simulink model "gm_inc_enc_v26_vnl"  (R2022b)
settings: Solver=FixedStepDiscrete  StartTime=0.0  StopTime=SimulationsDauer  RelTol=1e-3
undefined symbols (not defined in the file or in its folder): CW_CCW_Switch, d_axis_hit_CompareValue, DiscIntNeverNeededParam, f_ISR, IncPerTurn, inital_zero_speed_timeout, n_max, Offset_Position_elec, Offset_Position_mech, OmegaPerOverSampl, Periode, Phase_Delay_A, Phase_Delay_B, PolePair, QuadratureFactor, reciprocal_iterations, T_fpga, T_mech
libraries: simulink x25, hdlsllib x11, hdlmdlgenlib x4, dspsrcs4 x3, dspswit3 x2, spsEdgeDetectorLib x2, simulink_extras x1
(part 4 of 5)

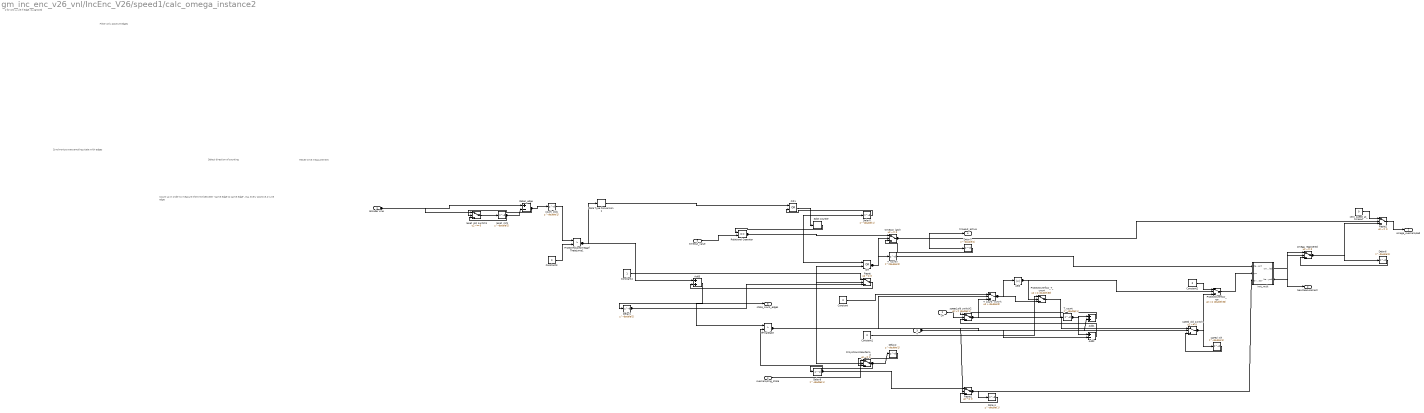
== system gm_inc_enc_v26_vnl/IncEnc_V26/speed1/calc_omega_instance2 ==
  note: Synchronize oversampling state with edges
  note: Filter only positive edges
  note: Select direction of counting
  note: 1 for one cycle if edge recognized
  note: Reset time measurement
  note: Count up in order to measure the time between "same edge to same edge", e.g. every positive A-Line edge
  Encoder Line : Inport  OutDataTypeStr=boolean  PortDimensions=1  SampleTime=1e-08
  Dir : Inport  Port=2  OutDataTypeStr=fixdt(1, 4, 0)  PortDimensions=1  SampleTime=1e-08
  T : Inport  Port=3  OutDataTypeStr=fixdt(1, 38, 32)  PortDimensions=1  SampleTime=1e-08
  oversampling_state : Inport  Port=4  OutDataTypeStr=uint16  PortDimensions=1  SampleTime=1e-08
  timeout_value : Inport  Port=5  OutDataTypeStr=uint32  PortDimensions=1  SampleTime=1e-08
  32bit counter : hdlsllib/Sources/HDL Counter  CountType=Free running  CountInit=0  CountStep=1  CountMax=inital_zero_speed_timeout  CountFromType=Initial value  CountFrom=0  CountResetPort=on  CountLoadPort=off  CountEnbPort=off  CountDirPort=off  CountHitOutputPort=off  CountDataType=Unsigned  CountWordLen=32  CountFracLen=0  CountSampTime=1
  ABS : Abs  SampleTime=1e-08  OutDataTypeStr=fixdt(1, 38, 32)  SaturateOnIntegerOverflow=off
  Add1 : Sum  AccumDataTypeStr=fixdt(1, 38, 32)  OutDataTypeStr=fixdt(1, 38, 32)  SampleTime=1e-08
  Add2 : Sum  Inputs=+-  AccumDataTypeStr=fixdt(1, 38, 32)  OutDataTypeStr=fixdt(1, 38, 32)  SampleTime=1e-08
  Add3 : Sum  AccumDataTypeStr=int16  OutDataTypeStr=int16  SampleTime=1e-08
  Constant : Constant  Value=0  OutDataTypeStr=fixdt(1, 38, 32)  SampleTime=1e-08
  Constant1 : Constant  Value=0  OutDataTypeStr=fixdt(1, 38, 32)  SampleTime=1e-08
  Constant2 : Constant  Value=0  OutDataTypeStr=fixdt(1, 38, 32)  SampleTime=1e-08
  Constant3 : Constant  Value=0  OutDataTypeStr=int8  SampleTime=1e-08
  Constant4 : Constant  OutDataTypeStr=int8  SampleTime=1e-08
  Data Type Conversion1 : DataTypeConversion  OutDataTypeStr=boolean  SampleTime=1e-08  SaturateOnIntegerOverflow=off  RndMeth=Floor
  Delay{1..6,8} (7 alike) : Delay  DelayLength=double(1)  InitialCondition=0  SampleTime=1e-08
  Detec_edge : Sum  Inputs=+-  AccumDataTypeStr=int8  OutDataTypeStr=int8  SampleTime=1e-08
  IfFinalState : RelationalOperator  Operator=>  OutDataTypeStr=boolean  SampleTime=1e-08  InputSameDT=off
  OR : Logic  Operator=OR  AllPortsSameDT=off  OutDataTypeStr=boolean  SampleTime=1e-08
  OR1 : Logic  Operator=OR  AllPortsSameDT=off  OutDataTypeStr=boolean  SampleTime=1e-08
  OnlyAllowInNewPeriod : Switch  Criteria=u2 ~= 0  Threshold=double(0)  OutDataTypeStr=uint16  SampleTime=1e-08  SaturateOnIntegerOverflow=off  InputSameDT=off
  ProtectOverflow_T_count : Switch  Threshold=double(30)  OutDataTypeStr=fixdt(1, 38, 32)  SampleTime=1e-08  SaturateOnIntegerOverflow=off  InputSameDT=off
  ProtectOverflow_rps : Switch  Threshold=double(30)  OutDataTypeStr=fixdt(1, 38, 32)  SampleTime=1e-08  SaturateOnIntegerOverflow=off  InputSameDT=off
  ProtectToUseOmegaIfThetaJump1 : RelationalOperator  Operator=>  OutDataTypeStr=fixdt(1,16,0)  SampleTime=1e-08  InputSameDT=off
  Relational Operator : RelationalOperator  Operator===  OutDataTypeStr=boolean  SampleTime=1e-08  InputSameDT=off
  Reset : Switch  Criteria=u2 ~= 0  Threshold=double(0)  OutDataTypeStr=fixdt(1, 24, 11)  SampleTime=1e-08  SaturateOnIntegerOverflow=off  InputSameDT=off
  Reset1 : Switch  Criteria=u2 ~= 0  Threshold=double(0)  OutDataTypeStr=uint16  SampleTime=1e-08  SaturateOnIntegerOverflow=off  InputSameDT=off
  Reset2 : Switch  Criteria=u2 ~= 0  Threshold=double(0)  OutDataTypeStr=fixdt(1, 24, 11)  SampleTime=1e-08  SaturateOnIntegerOverflow=off  InputSameDT=off
  T_count : Delay  DelayLength=double(1)  InitialCondition=0  SampleTime=1e-08
  T_count1 : Delay  DelayLength=double(2)  InitialCondition=0  SampleTime=1e-08
  T_count_switch : Switch  Criteria=u2 > Threshold  Threshold=double(0)  OutDataTypeStr=fixdt(1, 38, 32)  SampleTime=1e-08  SaturateOnIntegerOverflow=off  InputSameDT=off
  count_old1 : Delay  DelayLength=double(1)  InitialCondition=0  SampleTime=1e-08
  invt_mult : Subsystem
  omega_registered : Switch  Criteria=u2 ~= 0  Threshold=double(0)  OutDataTypeStr=fixdt(1, 24, 11)  SampleTime=1e-08  SaturateOnIntegerOverflow=off  InputSameDT=off
  reset_old1 : Delay  DelayLength=double(1)  InitialCondition=0  SampleTime=1e-08
  reset_old_switch1 : Switch  Criteria=u2 ~= 0  Threshold=double(0)  OutDataTypeStr=boolean  SampleTime=1e-08  SaturateOnIntegerOverflow=off  InputSameDT=off
  speed_old : Delay  DelayLength=double(1)  InitialCondition=0  SampleTime=1e-08
  speed_old_switch : Switch  Criteria=u2 ~= 0  Threshold=double(0)  OutDataTypeStr=fixdt(1, 38, 32)  SampleTime=1e-08  SaturateOnIntegerOverflow=off  InputSameDT=off
  speed_old_switch2 : Switch  Threshold=double(1)  OutDataTypeStr=fixdt(1, 38, 32)  SampleTime=1e-08  SaturateOnIntegerOverflow=off  InputSameDT=off
  timeout_latch : Switch  Criteria=u2 ~= 0  Threshold=double(0)  OutDataTypeStr=boolean  SampleTime=1e-08  SaturateOnIntegerOverflow=off  InputSameDT=off
  zero_speed_at_timeout : Constant  Value=0  OutDataTypeStr=fixdt(1, 24, 11)  SampleTime=1e-08
  omega_oversampled : Outport  SampleTime=1e-08  VectorParamsAs1DForOutWhenUnconnected=off
  NewMeasurement : Outport  Port=2  SampleTime=1e-08  VectorParamsAs1DForOutWhenUnconnected=off
  state_count_edges : Outport  Port=3  SampleTime=1e-08  VectorParamsAs1DForOutWhenUnconnected=off
  timeout_active : Outport  Port=4  OutDataTypeStr=boolean  SampleTime=1e-08  VectorParamsAs1DForOutWhenUnconnected=off
  wires:
  Encoder Line/1 -> Detec_edge/1, reset_old_switch1/1
  Dir/1 -> speed_old_switch2/2
  T/1 -> Add1/2, Add2/2
  oversampling_state/1 -> OnlyAllowInNewPeriod/1
  timeout_value/1 -> Relational Operator/2
  zero_speed_at_timeout/1 -> Reset2/1
  timeout_latch/1 -> Reset2/2, timeout_active/1, Delay3/1
  speed_old_switch2/1 -> T_count_switch/3, speed_old_switch/1
  speed_old_switch/1 -> ProtectOverflow_rps/3, speed_old/1
  omega_registered/1 -> Reset2/3, Delay6/1
  invt_mult/1(omega_oversampled) -> omega_registered/1
  invt_mult/2(New_Measurement_delayed) -> NewMeasurement/1, omega_registered/2
  count_old1/1 -> ProtectToUseOmegaIfThetaJump1/1
  T_count1/1 -> invt_mult/1(New_Measurement)
  Reset2/1 -> omega_oversampled/1
  Reset1/1 -> invt_mult/3(Oversampling Factor), Delay4/1
  Relational Operator/1 -> OR/1, Delay5/1, timeout_latch/1
  ProtectToUseOmegaIfThetaJump1/1 -> Data Type Conversion1/1, Add3/1
  ProtectOverflow_rps/1 -> invt_mult/2(rps)
  OR/1 -> T_count1/1, timeout_latch/2
  IfFinalState/1 -> OR/2, OnlyAllowInNewPeriod/2, Reset/2, T_count_switch/2, speed_old_switch/2, Reset1/2
  Detec_edge/1 -> count_old1/1, reset_old_switch1/2
  Delay8/1 -> IfFinalState/2, Reset1/1
  Delay1/1 -> state_count_edges/1, IfFinalState/1, Reset/3
  Data Type Conversion1/1 -> OR1/1
  Constant4/1 -> Reset/1
  Constant3/1 -> ProtectToUseOmegaIfThetaJump1/2
  Constant2/1 -> ProtectOverflow_rps/1
  Constant1/1 -> ProtectOverflow_T_count/1
  Constant/1 -> T_count_switch/1
  ABS/1 -> ProtectOverflow_rps/2, ProtectOverflow_T_count/2
  Delay6/1 -> omega_registered/3
  reset_old_switch1/1 -> reset_old1/1
  reset_old1/1 -> Detec_edge/2, reset_old_switch1/3
  OR1/1 -> 32bit counter/1
  Delay5/1 -> OR1/2
  32bit counter/1 -> Relational Operator/1
  Delay2/1 -> OnlyAllowInNewPeriod/3
  OnlyAllowInNewPeriod/1 -> Delay2/1, Delay8/1
  Reset/1 -> Add3/2
  Add3/1 -> Delay1/1
  Delay3/1 -> timeout_latch/3
  Add2/1 -> speed_old_switch2/3
  ProtectOverflow_T_count/1 -> T_count/1
  T_count/1 -> Add1/1, Add2/1
  Add1/1 -> speed_old_switch2/1
  T_count_switch/1 -> ABS/1, ProtectOverflow_T_count/3
  speed_old/1 -> speed_old_switch/3
  Delay4/1 -> Reset1/3

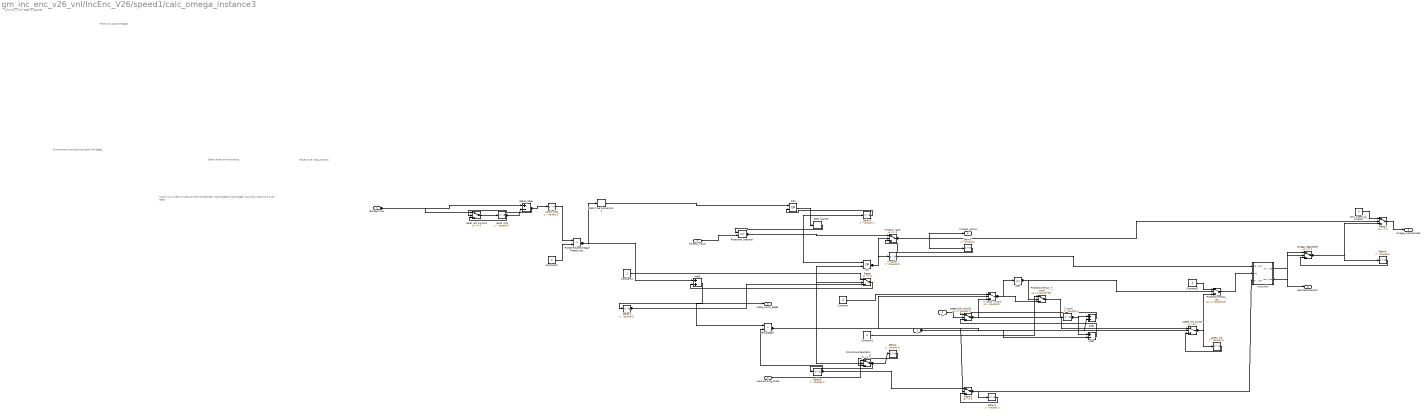
== system gm_inc_enc_v26_vnl/IncEnc_V26/speed1/calc_omega_instance3 ==
  note: Synchronize oversampling state with edges
  note: Filter only positive edges
  note: Select direction of counting
  note: 1 for one cycle if edge recognized
  note: Reset time measurement
  note: Count up in order to measure the time between "same edge to same edge", e.g. every positive A-Line edge
  Encoder Line : Inport  OutDataTypeStr=boolean  PortDimensions=1  SampleTime=1e-08
  Dir : Inport  Port=2  OutDataTypeStr=fixdt(1, 4, 0)  PortDimensions=1  SampleTime=1e-08
  T : Inport  Port=3  OutDataTypeStr=fixdt(1, 38, 32)  PortDimensions=1  SampleTime=1e-08
  oversampling_state : Inport  Port=4  OutDataTypeStr=uint16  PortDimensions=1  SampleTime=1e-08
  timeout_value : Inport  Port=5  OutDataTypeStr=uint32  PortDimensions=1  SampleTime=1e-08
  32bit counter : hdlsllib/Sources/HDL Counter  CountType=Free running  CountInit=0  CountStep=1  CountMax=inital_zero_speed_timeout  CountFromType=Initial value  CountFrom=0  CountResetPort=on  CountLoadPort=off  CountEnbPort=off  CountDirPort=off  CountHitOutputPort=off  CountDataType=Unsigned  CountWordLen=32  CountFracLen=0  CountSampTime=1
  ABS : Abs  SampleTime=1e-08  OutDataTypeStr=fixdt(1, 38, 32)  SaturateOnIntegerOverflow=off
  Add1 : Sum  AccumDataTypeStr=fixdt(1, 38, 32)  OutDataTypeStr=fixdt(1, 38, 32)  SampleTime=1e-08
  Add2 : Sum  Inputs=+-  AccumDataTypeStr=fixdt(1, 38, 32)  OutDataTypeStr=fixdt(1, 38, 32)  SampleTime=1e-08
  Add3 : Sum  AccumDataTypeStr=int16  OutDataTypeStr=int16  SampleTime=1e-08
  Constant : Constant  Value=0  OutDataTypeStr=fixdt(1, 38, 32)  SampleTime=1e-08
  Constant1 : Constant  Value=0  OutDataTypeStr=fixdt(1, 38, 32)  SampleTime=1e-08
  Constant2 : Constant  Value=0  OutDataTypeStr=fixdt(1, 38, 32)  SampleTime=1e-08
  Constant3 : Constant  Value=0  OutDataTypeStr=int8  SampleTime=1e-08
  Constant4 : Constant  OutDataTypeStr=int8  SampleTime=1e-08
  Data Type Conversion1 : DataTypeConversion  OutDataTypeStr=boolean  SampleTime=1e-08  SaturateOnIntegerOverflow=off  RndMeth=Floor
  Delay{1..6,8} (7 alike) : Delay  DelayLength=double(1)  InitialCondition=0  SampleTime=1e-08
  Detec_edge : Sum  Inputs=+-  AccumDataTypeStr=int8  OutDataTypeStr=int8  SampleTime=1e-08
  IfFinalState : RelationalOperator  Operator=>  OutDataTypeStr=boolean  SampleTime=1e-08  InputSameDT=off
  OR : Logic  Operator=OR  AllPortsSameDT=off  OutDataTypeStr=boolean  SampleTime=1e-08
  OR1 : Logic  Operator=OR  AllPortsSameDT=off  OutDataTypeStr=boolean  SampleTime=1e-08
  OnlyAllowInNewPeriod : Switch  Criteria=u2 ~= 0  Threshold=double(0)  OutDataTypeStr=uint16  SampleTime=1e-08  SaturateOnIntegerOverflow=off  InputSameDT=off
  ProtectOverflow_T_count : Switch  Threshold=double(30)  OutDataTypeStr=fixdt(1, 38, 32)  SampleTime=1e-08  SaturateOnIntegerOverflow=off  InputSameDT=off
  ProtectOverflow_rps : Switch  Threshold=double(30)  OutDataTypeStr=fixdt(1, 38, 32)  SampleTime=1e-08  SaturateOnIntegerOverflow=off  InputSameDT=off
  ProtectToUseOmegaIfThetaJump1 : RelationalOperator  Operator=>  OutDataTypeStr=fixdt(1,16,0)  SampleTime=1e-08  InputSameDT=off
  Relational Operator : RelationalOperator  Operator===  OutDataTypeStr=boolean  SampleTime=1e-08  InputSameDT=off
  Reset : Switch  Criteria=u2 ~= 0  Threshold=double(0)  OutDataTypeStr=fixdt(1, 24, 11)  SampleTime=1e-08  SaturateOnIntegerOverflow=off  InputSameDT=off
  Reset1 : Switch  Criteria=u2 ~= 0  Threshold=double(0)  OutDataTypeStr=uint16  SampleTime=1e-08  SaturateOnIntegerOverflow=off  InputSameDT=off
  Reset2 : Switch  Criteria=u2 ~= 0  Threshold=double(0)  OutDataTypeStr=fixdt(1, 24, 11)  SampleTime=1e-08  SaturateOnIntegerOverflow=off  InputSameDT=off
  T_count : Delay  DelayLength=double(1)  InitialCondition=0  SampleTime=1e-08
  T_count1 : Delay  DelayLength=double(2)  InitialCondition=0  SampleTime=1e-08
  T_count_switch : Switch  Criteria=u2 > Threshold  Threshold=double(0)  OutDataTypeStr=fixdt(1, 38, 32)  SampleTime=1e-08  SaturateOnIntegerOverflow=off  InputSameDT=off
  count_old1 : Delay  DelayLength=double(1)  InitialCondition=0  SampleTime=1e-08
  invt_mult : Subsystem
  omega_registered : Switch  Criteria=u2 ~= 0  Threshold=double(0)  OutDataTypeStr=fixdt(1, 24, 11)  SampleTime=1e-08  SaturateOnIntegerOverflow=off  InputSameDT=off
  reset_old1 : Delay  DelayLength=double(1)  InitialCondition=0  SampleTime=1e-08
  reset_old_switch1 : Switch  Criteria=u2 ~= 0  Threshold=double(0)  OutDataTypeStr=boolean  SampleTime=1e-08  SaturateOnIntegerOverflow=off  InputSameDT=off
  speed_old : Delay  DelayLength=double(1)  InitialCondition=0  SampleTime=1e-08
  speed_old_switch : Switch  Criteria=u2 ~= 0  Threshold=double(0)  OutDataTypeStr=fixdt(1, 38, 32)  SampleTime=1e-08  SaturateOnIntegerOverflow=off  InputSameDT=off
  speed_old_switch2 : Switch  Threshold=double(1)  OutDataTypeStr=fixdt(1, 38, 32)  SampleTime=1e-08  SaturateOnIntegerOverflow=off  InputSameDT=off
  timeout_latch : Switch  Criteria=u2 ~= 0  Threshold=double(0)  OutDataTypeStr=boolean  SampleTime=1e-08  SaturateOnIntegerOverflow=off  InputSameDT=off
  zero_speed_at_timeout : Constant  Value=0  OutDataTypeStr=fixdt(1, 24, 11)  SampleTime=1e-08
  omega_oversampled : Outport  SampleTime=1e-08  VectorParamsAs1DForOutWhenUnconnected=off
  NewMeasurement : Outport  Port=2  SampleTime=1e-08  VectorParamsAs1DForOutWhenUnconnected=off
  state_count_edges : Outport  Port=3  SampleTime=1e-08  VectorParamsAs1DForOutWhenUnconnected=off
  timeout_active : Outport  Port=4  OutDataTypeStr=boolean  SampleTime=1e-08  VectorParamsAs1DForOutWhenUnconnected=off
  wires:
  Encoder Line/1 -> Detec_edge/1, reset_old_switch1/1
  Dir/1 -> speed_old_switch2/2
  T/1 -> Add1/2, Add2/2
  oversampling_state/1 -> OnlyAllowInNewPeriod/1
  timeout_value/1 -> Relational Operator/2
  zero_speed_at_timeout/1 -> Reset2/1
  timeout_latch/1 -> Reset2/2, timeout_active/1, Delay3/1
  speed_old_switch2/1 -> T_count_switch/3, speed_old_switch/1
  speed_old_switch/1 -> ProtectOverflow_rps/3, speed_old/1
  omega_registered/1 -> Reset2/3, Delay6/1
  invt_mult/1(omega_oversampled) -> omega_registered/1
  invt_mult/2(New_Measurement_delayed) -> NewMeasurement/1, omega_registered/2
  count_old1/1 -> ProtectToUseOmegaIfThetaJump1/1
  T_count1/1 -> invt_mult/1(New_Measurement)
  Reset2/1 -> omega_oversampled/1
  Reset1/1 -> invt_mult/3(Oversampling Factor), Delay4/1
  Relational Operator/1 -> OR/1, Delay5/1, timeout_latch/1
  ProtectToUseOmegaIfThetaJump1/1 -> Data Type Conversion1/1, Add3/1
  ProtectOverflow_rps/1 -> invt_mult/2(rps)
  OR/1 -> T_count1/1, timeout_latch/2
  IfFinalState/1 -> OR/2, OnlyAllowInNewPeriod/2, Reset/2, T_count_switch/2, speed_old_switch/2, Reset1/2
  Detec_edge/1 -> count_old1/1, reset_old_switch1/2
  Delay8/1 -> IfFinalState/2, Reset1/1
  Delay1/1 -> state_count_edges/1, IfFinalState/1, Reset/3
  Data Type Conversion1/1 -> OR1/1
  Constant4/1 -> Reset/1
  Constant3/1 -> ProtectToUseOmegaIfThetaJump1/2
  Constant2/1 -> ProtectOverflow_rps/1
  Constant1/1 -> ProtectOverflow_T_count/1
  Constant/1 -> T_count_switch/1
  ABS/1 -> ProtectOverflow_rps/2, ProtectOverflow_T_count/2
  Delay6/1 -> omega_registered/3
  reset_old_switch1/1 -> reset_old1/1
  reset_old1/1 -> Detec_edge/2, reset_old_switch1/3
  OR1/1 -> 32bit counter/1
  Delay5/1 -> OR1/2
  32bit counter/1 -> Relational Operator/1
  Delay2/1 -> OnlyAllowInNewPeriod/3
  OnlyAllowInNewPeriod/1 -> Delay2/1, Delay8/1
  Reset/1 -> Add3/2
  Add3/1 -> Delay1/1
  Delay3/1 -> timeout_latch/3
  Add2/1 -> speed_old_switch2/3
  ProtectOverflow_T_count/1 -> T_count/1
  T_count/1 -> Add1/1, Add2/1
  Add1/1 -> speed_old_switch2/1
  T_count_switch/1 -> ABS/1, ProtectOverflow_T_count/3
  speed_old/1 -> speed_old_switch/3
  Delay4/1 -> Reset1/3

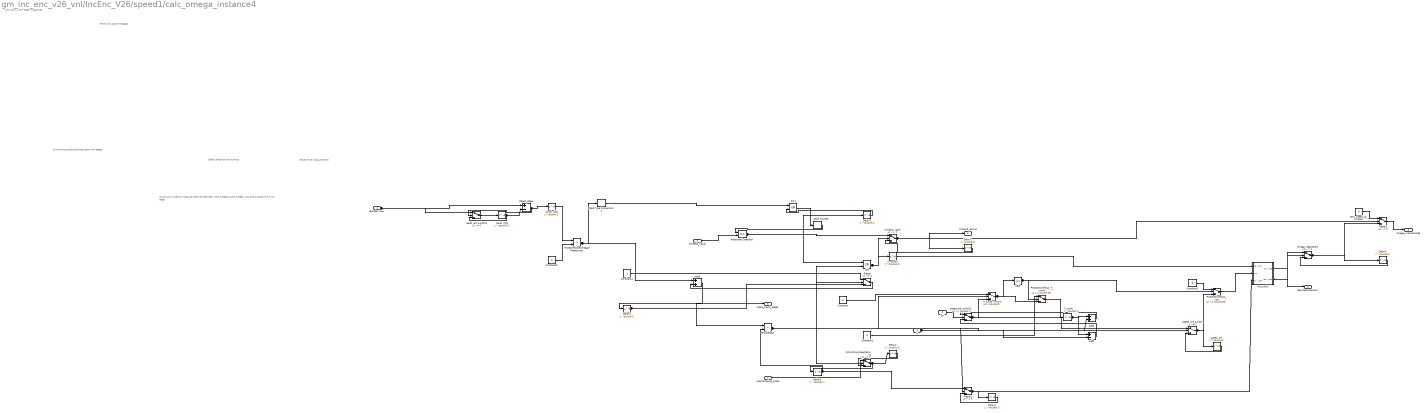
== system gm_inc_enc_v26_vnl/IncEnc_V26/speed1/calc_omega_instance4 ==
  note: Count up in order to measure the time between "same edge to same edge", e.g. every positive A-Line edge
  note: Reset time measurement
  note: 1 for one cycle if edge recognized
  note: Select direction of counting
  note: Filter only positive edges
  note: Synchronize oversampling state with edges
  Encoder Line : Inport  OutDataTypeStr=boolean  PortDimensions=1  SampleTime=1e-08
  Dir : Inport  Port=2  OutDataTypeStr=fixdt(1, 4, 0)  PortDimensions=1  SampleTime=1e-08
  T : Inport  Port=3  OutDataTypeStr=fixdt(1, 38, 32)  PortDimensions=1  SampleTime=1e-08
  oversampling_state : Inport  Port=4  OutDataTypeStr=uint16  PortDimensions=1  SampleTime=1e-08
  timeout_value : Inport  Port=5  OutDataTypeStr=uint32  PortDimensions=1  SampleTime=1e-08
  32bit counter : hdlsllib/Sources/HDL Counter  CountType=Free running  CountInit=0  CountStep=1  CountMax=inital_zero_speed_timeout  CountFromType=Initial value  CountFrom=0  CountResetPort=on  CountLoadPort=off  CountEnbPort=off  CountDirPort=off  CountHitOutputPort=off  CountDataType=Unsigned  CountWordLen=32  CountFracLen=0  CountSampTime=1
  ABS : Abs  SampleTime=1e-08  OutDataTypeStr=fixdt(1, 38, 32)  SaturateOnIntegerOverflow=off
  Add1 : Sum  AccumDataTypeStr=fixdt(1, 38, 32)  OutDataTypeStr=fixdt(1, 38, 32)  SampleTime=1e-08
  Add2 : Sum  Inputs=+-  AccumDataTypeStr=fixdt(1, 38, 32)  OutDataTypeStr=fixdt(1, 38, 32)  SampleTime=1e-08
  Add3 : Sum  AccumDataTypeStr=int16  OutDataTypeStr=int16  SampleTime=1e-08
  Constant : Constant  Value=0  OutDataTypeStr=fixdt(1, 38, 32)  SampleTime=1e-08
  Constant1 : Constant  Value=0  OutDataTypeStr=fixdt(1, 38, 32)  SampleTime=1e-08
  Constant2 : Constant  Value=0  OutDataTypeStr=fixdt(1, 38, 32)  SampleTime=1e-08
  Constant3 : Constant  Value=0  OutDataTypeStr=int8  SampleTime=1e-08
  Constant4 : Constant  OutDataTypeStr=int8  SampleTime=1e-08
  Data Type Conversion1 : DataTypeConversion  OutDataTypeStr=boolean  SampleTime=1e-08  SaturateOnIntegerOverflow=off  RndMeth=Floor
  Delay{1..6,8} (7 alike) : Delay  DelayLength=double(1)  InitialCondition=0  SampleTime=1e-08
  Detec_edge : Sum  Inputs=+-  AccumDataTypeStr=int8  OutDataTypeStr=int8  SampleTime=1e-08
  IfFinalState : RelationalOperator  Operator=>  OutDataTypeStr=boolean  SampleTime=1e-08  InputSameDT=off
  OR : Logic  Operator=OR  AllPortsSameDT=off  OutDataTypeStr=boolean  SampleTime=1e-08
  OR1 : Logic  Operator=OR  AllPortsSameDT=off  OutDataTypeStr=boolean  SampleTime=1e-08
  OnlyAllowInNewPeriod : Switch  Criteria=u2 ~= 0  Threshold=double(0)  OutDataTypeStr=uint16  SampleTime=1e-08  SaturateOnIntegerOverflow=off  InputSameDT=off
  ProtectOverflow_T_count : Switch  Threshold=double(30)  OutDataTypeStr=fixdt(1, 38, 32)  SampleTime=1e-08  SaturateOnIntegerOverflow=off  InputSameDT=off
  ProtectOverflow_rps : Switch  Threshold=double(30)  OutDataTypeStr=fixdt(1, 38, 32)  SampleTime=1e-08  SaturateOnIntegerOverflow=off  InputSameDT=off
  ProtectToUseOmegaIfThetaJump1 : RelationalOperator  Operator=>  OutDataTypeStr=fixdt(1,16,0)  SampleTime=1e-08  InputSameDT=off
  Relational Operator : RelationalOperator  Operator===  OutDataTypeStr=boolean  SampleTime=1e-08  InputSameDT=off
  Reset : Switch  Criteria=u2 ~= 0  Threshold=double(0)  OutDataTypeStr=fixdt(1, 24, 11)  SampleTime=1e-08  SaturateOnIntegerOverflow=off  InputSameDT=off
  Reset1 : Switch  Criteria=u2 ~= 0  Threshold=double(0)  OutDataTypeStr=uint16  SampleTime=1e-08  SaturateOnIntegerOverflow=off  InputSameDT=off
  Reset2 : Switch  Criteria=u2 ~= 0  Threshold=double(0)  OutDataTypeStr=fixdt(1, 24, 11)  SampleTime=1e-08  SaturateOnIntegerOverflow=off  InputSameDT=off
  T_count : Delay  DelayLength=double(1)  InitialCondition=0  SampleTime=1e-08
  T_count1 : Delay  DelayLength=double(2)  InitialCondition=0  SampleTime=1e-08
  T_count_switch : Switch  Criteria=u2 > Threshold  Threshold=double(0)  OutDataTypeStr=fixdt(1, 38, 32)  SampleTime=1e-08  SaturateOnIntegerOverflow=off  InputSameDT=off
  count_old1 : Delay  DelayLength=double(1)  InitialCondition=0  SampleTime=1e-08
  invt_mult : Subsystem
  omega_registered : Switch  Criteria=u2 ~= 0  Threshold=double(0)  OutDataTypeStr=fixdt(1, 24, 11)  SampleTime=1e-08  SaturateOnIntegerOverflow=off  InputSameDT=off
  reset_old1 : Delay  DelayLength=double(1)  InitialCondition=0  SampleTime=1e-08
  reset_old_switch1 : Switch  Criteria=u2 ~= 0  Threshold=double(0)  OutDataTypeStr=boolean  SampleTime=1e-08  SaturateOnIntegerOverflow=off  InputSameDT=off
  speed_old : Delay  DelayLength=double(1)  InitialCondition=0  SampleTime=1e-08
  speed_old_switch : Switch  Criteria=u2 ~= 0  Threshold=double(0)  OutDataTypeStr=fixdt(1, 38, 32)  SampleTime=1e-08  SaturateOnIntegerOverflow=off  InputSameDT=off
  speed_old_switch2 : Switch  Threshold=double(1)  OutDataTypeStr=fixdt(1, 38, 32)  SampleTime=1e-08  SaturateOnIntegerOverflow=off  InputSameDT=off
  timeout_latch : Switch  Criteria=u2 ~= 0  Threshold=double(0)  OutDataTypeStr=boolean  SampleTime=1e-08  SaturateOnIntegerOverflow=off  InputSameDT=off
  zero_speed_at_timeout : Constant  Value=0  OutDataTypeStr=fixdt(1, 24, 11)  SampleTime=1e-08
  omega_oversampled : Outport  SampleTime=1e-08  VectorParamsAs1DForOutWhenUnconnected=off
  NewMeasurement : Outport  Port=2  SampleTime=1e-08  VectorParamsAs1DForOutWhenUnconnected=off
  state_count_edges : Outport  Port=3  SampleTime=1e-08  VectorParamsAs1DForOutWhenUnconnected=off
  timeout_active : Outport  Port=4  OutDataTypeStr=boolean  SampleTime=1e-08  VectorParamsAs1DForOutWhenUnconnected=off
  wires:
  Delay4/1 -> Reset1/3
  speed_old/1 -> speed_old_switch/3
  T_count_switch/1 -> ProtectOverflow_T_count/3, ABS/1
  Add1/1 -> speed_old_switch2/1
  T_count/1 -> Add2/1, Add1/1
  ProtectOverflow_T_count/1 -> T_count/1
  Add2/1 -> speed_old_switch2/3
  Delay3/1 -> timeout_latch/3
  Add3/1 -> Delay1/1
  Reset/1 -> Add3/2
  OnlyAllowInNewPeriod/1 -> Delay8/1, Delay2/1
  Delay2/1 -> OnlyAllowInNewPeriod/3
  32bit counter/1 -> Relational Operator/1
  Delay5/1 -> OR1/2
  OR1/1 -> 32bit counter/1
  reset_old1/1 -> reset_old_switch1/3, Detec_edge/2
  reset_old_switch1/1 -> reset_old1/1
  Delay6/1 -> omega_registered/3
  ABS/1 -> ProtectOverflow_T_count/2, ProtectOverflow_rps/2
  Constant/1 -> T_count_switch/1
  Constant1/1 -> ProtectOverflow_T_count/1
  Constant2/1 -> ProtectOverflow_rps/1
  Constant3/1 -> ProtectToUseOmegaIfThetaJump1/2
  Constant4/1 -> Reset/1
  Data Type Conversion1/1 -> OR1/1
  Delay1/1 -> Reset/3, IfFinalState/1, state_count_edges/1
  Delay8/1 -> Reset1/1, IfFinalState/2
  Detec_edge/1 -> reset_old_switch1/2, count_old1/1
  IfFinalState/1 -> Reset1/2, speed_old_switch/2, T_count_switch/2, Reset/2, OnlyAllowInNewPeriod/2, OR/2
  OR/1 -> timeout_latch/2, T_count1/1
  ProtectOverflow_rps/1 -> invt_mult/2(rps)
  ProtectToUseOmegaIfThetaJump1/1 -> Add3/1, Data Type Conversion1/1
  Relational Operator/1 -> timeout_latch/1, Delay5/1, OR/1
  Reset1/1 -> Delay4/1, invt_mult/3(Oversampling Factor)
  Reset2/1 -> omega_oversampled/1
  T_count1/1 -> invt_mult/1(New_Measurement)
  count_old1/1 -> ProtectToUseOmegaIfThetaJump1/1
  invt_mult/2(New_Measurement_delayed) -> omega_registered/2, NewMeasurement/1
  invt_mult/1(omega_oversampled) -> omega_registered/1
  omega_registered/1 -> Delay6/1, Reset2/3
  speed_old_switch/1 -> speed_old/1, ProtectOverflow_rps/3
  speed_old_switch2/1 -> speed_old_switch/1, T_count_switch/3
  timeout_latch/1 -> Delay3/1, timeout_active/1, Reset2/2
  zero_speed_at_timeout/1 -> Reset2/1
  timeout_value/1 -> Relational Operator/2
  oversampling_state/1 -> OnlyAllowInNewPeriod/1
  T/1 -> Add2/2, Add1/2
  Dir/1 -> speed_old_switch2/2
  Encoder Line/1 -> reset_old_switch1/1, Detec_edge/1

== system gm_inc_enc_v26_vnl/IncEnc_V26_vnl/Counter_Theta_el_wOffset/Subsystem ==
  Add1 : Sum  AccumDataTypeStr=int16  OutDataTypeStr=int16
  Constant3 : Constant  Value=0  OutDataTypeStr=int16  SampleTime=-1
  Generate_Increment : Subsystem
  Resett_switch2 : Switch  Criteria=u2 ~= 0  OutDataTypeStr=int16  SaturateOnIntegerOverflow=off  InputSameDT=off
  reset_old6 : Delay  DelayLength=1
  speed_old_switch1 : Switch  Criteria=u2 ~= 0  SaturateOnIntegerOverflow=off  InputSameDT=off
  wires:
  speed_old_switch1/1 -> Add1/1
  Add1/1 -> Resett_switch2/3
  reset_old6/1 -> Resett_switch2/1
  ? -> Generate_Increment/1(Dir_in)
  Constant3/1 -> speed_old_switch1/3
  Resett_switch2/1 -> ?
  Generate_Increment/1(Increment) -> speed_old_switch1/1
  ? -> Add1/2
  ? -> reset_old6/1
  ? -> Resett_switch2/2
  ? -> speed_old_switch1/2

== system gm_inc_enc_v26_vnl/IncEnc_V26_vnl/Counter_position_wOffset/Subsystem ==
  Add1 : Sum  AccumDataTypeStr=int16  OutDataTypeStr=int16
  Constant3 : Constant  Value=0  OutDataTypeStr=int16  SampleTime=-1
  Generate_Increment : Subsystem
  Resett_switch2 : Switch  Criteria=u2 ~= 0  OutDataTypeStr=int16  SaturateOnIntegerOverflow=off  InputSameDT=off
  reset_old6 : Delay  DelayLength=1
  speed_old_switch1 : Switch  Criteria=u2 ~= 0  SaturateOnIntegerOverflow=off  InputSameDT=off
  wires:
  ? -> speed_old_switch1/2
  ? -> Resett_switch2/2
  ? -> reset_old6/1
  ? -> Add1/2
  Generate_Increment/1(Increment) -> speed_old_switch1/1
  Resett_switch2/1 -> ?
  Constant3/1 -> speed_old_switch1/3
  ? -> Generate_Increment/1(Dir_in)
  reset_old6/1 -> Resett_switch2/1
  Add1/1 -> Resett_switch2/3
  speed_old_switch1/1 -> Add1/1

== system gm_inc_enc_v26_vnl/IncEnc_V26_vnl/speed1/Average ==
  note: moving average of 4 last measurements, which in total results in a moving average of the last 8 samples
  note: average 4 parallel measurements
  "OmegaIn " : Inport
  NewMeasurement : Inport  Port=2
  DelayToCompensate_sum : Delay  DelayLength=1
  Demux2 : Demux
  Gain : Gain  Gain=1/4  OutDataTypeStr=fixdt(1,24,11)
  Gain1 : Gain  Gain=1/4  OutDataTypeStr=fixdt(1,24,11)
  Sum of Elements{1..6} (6 alike) : Sum  Inputs=2
  Unit Delay Enabled Synchronous : hdlsllib/Discrete/Unit Delay Enabled Synchronous  InitialCondition=0  SampleTime=-1
  Unit Delay Enabled Synchronous1 : hdlsllib/Discrete/Unit Delay Enabled Synchronous  InitialCondition=0  SampleTime=-1
  Unit Delay Enabled Synchronous2 : hdlsllib/Discrete/Unit Delay Enabled Synchronous  InitialCondition=0  SampleTime=-1
  delay : Delay  DelayLength=1
  delay1 : Delay  DelayLength=1
  Omega : Outport  VectorParamsAs1DForOutWhenUnconnected=off
  OmegaOut_MA_N4 : Outport  Port=2  VectorParamsAs1DForOutWhenUnconnected=off
  wires:
  "OmegaIn "/1 -> Demux2/1  "x(k)"
  Sum of Elements6/1 -> Gain1/1
  Gain1/1 -> DelayToCompensate_sum/1  "omega summed 1/4"
  Demux2/2 -> Sum of Elements4/2
  Sum of Elements4/1 -> Sum of Elements6/1
  Sum of Elements5/1 -> Sum of Elements6/2
  Demux2/1 -> Sum of Elements4/1
  Demux2/3 -> Sum of Elements5/1
  Demux2/4 -> Sum of Elements5/2
  Unit Delay Enabled Synchronous1/1 -> Sum of Elements2/1, Unit Delay Enabled Synchronous2/1  "omega_delay2"
  delay/1 -> Unit Delay Enabled Synchronous2/2, Unit Delay Enabled Synchronous1/2, Unit Delay Enabled Synchronous/2  "enable_delayed"
  Sum of Elements2/1 -> Sum of Elements3/2
  NewMeasurement/1 -> delay/1
  delay1/1 -> Sum of Elements1/1  "x(k)_1delayed"
  Unit Delay Enabled Synchronous2/1 -> Sum of Elements2/2  "omega_delay3"
  Sum of Elements3/1 -> Gain/1
  Sum of Elements1/1 -> Sum of Elements3/1
  Unit Delay Enabled Synchronous/1 -> Unit Delay Enabled Synchronous1/1, Sum of Elements1/2  "omega_delay1"
  DelayToCompensate_sum/1 -> Omega/1, delay1/1, Unit Delay Enabled Synchronous/1  "x(k)"
  Gain/1 -> OmegaOut_MA_N4/1  "omega moving average"

== system gm_inc_enc_v26_vnl/IncEnc_V26_vnl/speed1/OS_factor_logic ==
  new_transisiton : Inport  PortDimensions=4
  Allow_ToCheckOversampling : Inport  Port=2
  state_edges : Inport  Port=3
  omega : Inport  Port=4
  OverSamplOmega : Inport  Port=5
  Abs : Abs  SaturateOnIntegerOverflow=off
  Constant : Constant  Commented=on  Value=[0,0,0,0]  OutDataTypeStr=boolean  SampleTime=T_fpga
  Data Type Conversion1 : DataTypeConversion  OutDataTypeStr=uint16  SaturateOnIntegerOverflow=off  RndMeth=Floor
  Delay1 : Delay  DelayLength=1  InitialCondition=0
  Delay6 : Delay  DelayLength=1  InitialCondition=0
  Delay7 : Delay  DelayLength=1  InitialCondition=1
  Sum : Sum  Inputs=+|-  AccumDataTypeStr=uint16
  align_oversamples : MATLAB Function  TreatAsAtomicUnit=on
  oversample_factor : MATLAB Function  TreatAsAtomicUnit=on
  oversampling_adjusted : Outport  PortDimensions=4
  oversampling_state : Outport  Port=2
  wires:
  Delay1/1 -> Sum/2
  Sum/1 -> oversampling_adjusted/1
  state_edges/1 -> align_oversamples/3(states)  "states"
  new_transisiton/1 -> align_oversamples/2(new_transition)  "new_transistions"
  align_oversamples/1(delay_output) -> Delay1/1  "delay_output"
  Data Type Conversion1/1 -> oversampling_state/1
  Delay7/1 -> Data Type Conversion1/1, oversample_factor/4(state), align_oversamples/1(oversampling_factor), Sum/1
  Allow_ToCheckOversampling/1 -> oversample_factor/1(AllowCheckOverSampl)  "Allow_ToCheckOversampling"
  Abs/1 -> oversample_factor/2(ReadBack_Omega)
  Delay6/1 -> oversample_factor/5(InternalOmega)
  oversample_factor/2(InternalOmega_Out) -> Delay6/1
  omega/1 -> Abs/1
  oversample_factor/1(state_Out) -> Delay7/1  "oversampling state Out"
  OverSamplOmega/1 -> oversample_factor/3(OverSamplOmega)

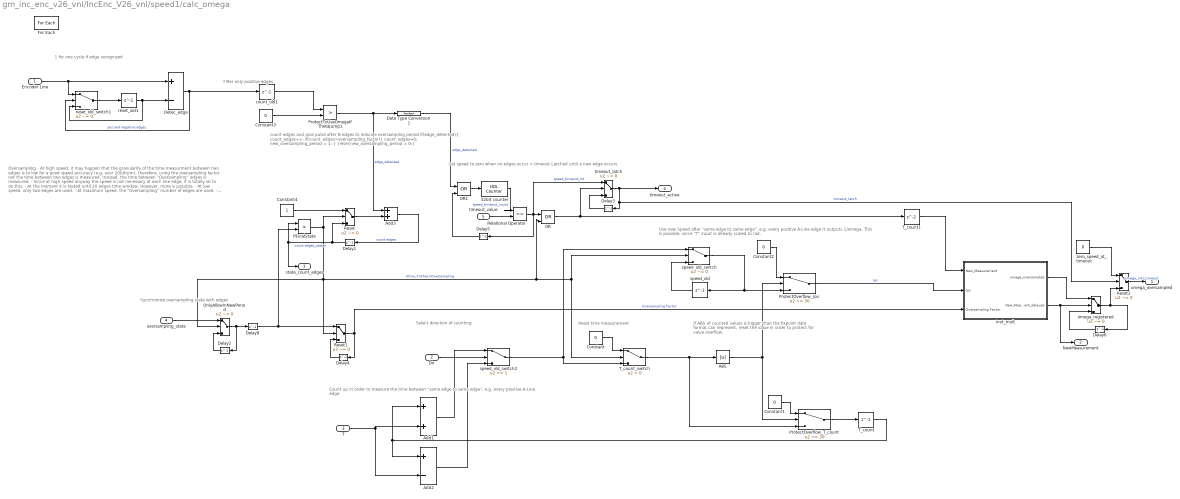
== system gm_inc_enc_v26_vnl/IncEnc_V26_vnl/speed1/calc_omega ==
  note: Set speed to zero when no edges occur = timeout
      | Latched until a new edge occurs
  note: Synchronize oversampling state with edges
  note: count edges and give pulse after N edges to indicate oversampling period
      | if(edge_detected){
      | 	count_edges++;
      | 	if(count_edges>oversampling_factor){
      | 		count_edges=0;
      | 		new_oversampling_period = 1;
      | 	}
      | }else{new_oversampling_period = 0;}
  note: Filter only positive edges
  note: If ABS of counted values is bigger than the
      | fixpoint data format can represent, reset the
      | value in order to protect for value overflow.
  note: Select direction of counting
  note: Use new Speed after "same edge to same edge", e.g. every positive A-Line edge
      | It outputs 1/omega. This is possible, since "T" input is already scaled to rad.
  note: 1 for one cycle if edge recognized
  note: Reset time measurement
  note: Count up in order to measure the time between "same edge to same edge", e.g. every positive A-Line edge
  note: Oversampling
      | - At high speed, it may happen that the granularity of the time measurment between
      | two edges is to low for a good speed accuracy (e.g. over 2000rpm), therefore, using
      | the oversampling factor, not the time between two edges is measured. Instead, the
      | time between "Oversampling" edges is measured.
      | - Since at high speed anyway the speed is not necessary at each line edge,
      |  it is totally ok to do this.
      | - At the moment it is tested until 20 edges time window. However, more is possible.
      | - At low speed, only two edges are used.
      | - At maximum speed, the "Oversampling" number of edges are used.
      | - Between them, a linear factor is used.
      | - Using the OverSampling number also at low speed is not possible,
      |  since the fixpoint range must be quite high! (fixdt(1,36,30) is used at the moment)
  Encoder Line : Inport  Partition=on  PartitionDimension=1  PartitionWidth=1  PartitionOffset=0
  Dir : Inport  Port=2
  T : Inport  Port=3
  oversampling_state : Inport  Port=4  Partition=on  PartitionDimension=1  PartitionWidth=1  PartitionOffset=0
  timeout_value : Inport  Port=5  OutDataTypeStr=uint32
  32bit counter : hdlsllib/Sources/HDL Counter  CountType=Free running  CountInit=0  CountStep=1  CountMax=inital_zero_speed_timeout  CountFromType=Initial value  CountFrom=0  CountResetPort=on  CountLoadPort=off  CountEnbPort=off  CountDirPort=off  CountHitOutputPort=off  CountDataType=Unsigned  CountWordLen=32  CountFracLen=0  CountSampTime=1
  ABS : Abs  SaturateOnIntegerOverflow=off
  Add1 : Sum  OutDataTypeStr=Inherit: Same as first input
  Add2 : Sum  Inputs=+-  OutDataTypeStr=Inherit: Same as first input
  Add3 : Sum  OutDataTypeStr=Inherit: Same as accumulator
  Constant : Constant  Value=0  OutDataTypeStr=fixdt(1,38,32)  SampleTime=-1
  Constant1 : Constant  Value=0  OutDataTypeStr=fixdt(1,38,32)  SampleTime=-1
  Constant2 : Constant  Value=0  OutDataTypeStr=fixdt(1,38,32)  SampleTime=-1
  Constant3 : Constant  Value=0  OutDataTypeStr=int8  SampleTime=-1
  Constant4 : Constant  OutDataTypeStr=int8  SampleTime=-1
  Data Type Conversion1 : DataTypeConversion  OutDataTypeStr=boolean  SaturateOnIntegerOverflow=off  RndMeth=Floor
  Delay{1..6,8} (7 alike) : Delay  DelayLength=1  InitialCondition=0
  Detec_edge : Sum  Inputs=+-  AccumDataTypeStr=int8  OutDataTypeStr=int8
  For Each : ForEach  DisableCoverage=on
  IfFinalState : RelationalOperator  Operator=>  OutDataTypeStr=boolean  InputSameDT=off
  OR : Logic  Operator=OR  IconShape=distinctive  AllPortsSameDT=off  OutDataTypeStr=boolean
  OR1 : Logic  Operator=OR  IconShape=distinctive  AllPortsSameDT=off  OutDataTypeStr=boolean
  OnlyAllowInNewPeriod : Switch  Criteria=u2 ~= 0  Threshold=0.5  OutDataTypeStr=fixdt(0,16,0)  SaturateOnIntegerOverflow=off  InputSameDT=off
  ProtectOverflow_T_count : Switch  Threshold=30  SaturateOnIntegerOverflow=off  InputSameDT=off
  ProtectOverflow_rps : Switch  Threshold=30  OutDataTypeStr=fixdt(1,38,32)  SaturateOnIntegerOverflow=off  InputSameDT=off
  ProtectToUseOmegaIfThetaJump1 : RelationalOperator  Operator=>  OutDataTypeStr=fixdt(1,16)  InputSameDT=off
  Relational Operator : RelationalOperator  Operator===  OutDataTypeStr=boolean  RndMeth=Simplest  InputSameDT=off
  Reset : Switch  Criteria=u2 ~= 0  Threshold=0.5  OutDataTypeStr=fixdt(1,24,11)  SaturateOnIntegerOverflow=off  InputSameDT=off
  Reset1 : Switch  Criteria=u2 ~= 0  Threshold=0.5  OutDataTypeStr=Inherit: Inherit via back propagation  SaturateOnIntegerOverflow=off  InputSameDT=off
  Reset2 : Switch  Criteria=u2 ~= 0  Threshold=0.5  OutDataTypeStr=Inherit: Inherit via back propagation  SaturateOnIntegerOverflow=off  InputSameDT=off
  T_count : Delay  DelayLength=1
  T_count1 : Delay
  T_count_switch : Switch  Criteria=u2 > Threshold  SaturateOnIntegerOverflow=off  InputSameDT=off
  count_old1 : Delay  DelayLength=1
  invt_mult : Subsystem
  omega_registered : Switch  Criteria=u2 ~= 0  Threshold=0.5  SaturateOnIntegerOverflow=off  InputSameDT=off
  reset_old1 : Delay  DelayLength=1
  reset_old_switch1 : Switch  Criteria=u2 ~= 0  SaturateOnIntegerOverflow=off  InputSameDT=off
  speed_old : Delay  DelayLength=1
  speed_old_switch : Switch  Criteria=u2 ~= 0  OutDataTypeStr=fixdt(1,38,32)  SaturateOnIntegerOverflow=off  InputSameDT=off
  speed_old_switch2 : Switch  Threshold=1  SaturateOnIntegerOverflow=off  InputSameDT=off
  timeout_latch : Switch  Criteria=u2 ~= 0  Threshold=0.5  OutDataTypeStr=Inherit: Inherit via back propagation  SaturateOnIntegerOverflow=off  InputSameDT=off
  zero_speed_at_timeout : Constant  Value=0  OutDataTypeStr=fixdt(1,24,11)  SampleTime=-1
  omega_oversampled : Outport  ConcatenationDimension=1  VectorParamsAs1DForOutWhenUnconnected=off
  NewMeasurement : Outport  Port=2  ConcatenationDimension=1  VectorParamsAs1DForOutWhenUnconnected=off
  state_count_edges : Outport  Port=3  ConcatenationDimension=1  VectorParamsAs1DForOutWhenUnconnected=off
  timeout_active : Outport  Port=4  OutDataTypeStr=boolean  ConcatenationDimension=1  VectorParamsAs1DForOutWhenUnconnected=off
  wires:
  T_count1/1 -> invt_mult/1(New_Measurement)
  invt_mult/2(New_Measurement_delayed) -> omega_registered/2, NewMeasurement/1
  invt_mult/1(omega_oversampled) -> omega_registered/1
  ProtectOverflow_rps/1 -> invt_mult/2(rps)  "rps"
  OR/1 -> timeout_latch/2, T_count1/1
  Delay6/1 -> omega_registered/3
  omega_registered/1 -> Delay6/1, Reset2/3
  Delay5/1 -> OR1/2
  OR1/1 -> 32bit counter/1
  32bit counter/1 -> Relational Operator/1  "speed_timeout_count"
  timeout_value/1 -> Relational Operator/2
  Data Type Conversion1/1 -> OR1/1  "edge_detected"
  Delay3/1 -> timeout_latch/3
  timeout_latch/1 -> Reset2/2, Delay3/1, timeout_active/1  "timeout_latch"
  Reset2/1 -> omega_oversampled/1  "omega_inkl_timeout"
  zero_speed_at_timeout/1 -> Reset2/1
  Relational Operator/1 -> timeout_latch/1, OR/1, Delay5/1  "speed_timeout_hit"
  ProtectToUseOmegaIfThetaJump1/1 -> Data Type Conversion1/1, Add3/1  "edge_detected"
  Delay8/1 -> IfFinalState/2, Reset1/1
  Delay4/1 -> Reset1/3
  oversampling_state/1 -> OnlyAllowInNewPeriod/1
  Delay2/1 -> OnlyAllowInNewPeriod/3
  Reset1/1 -> Delay4/1, invt_mult/3(Oversampling Factor)  "Oversampling Factor"
  Constant4/1 -> Reset/1
  Reset/1 -> Add3/2
  Add3/1 -> Delay1/1  "count edges"
  Delay1/1 -> IfFinalState/1, state_count_edges/1, Reset/3  "count edges_states"
  OnlyAllowInNewPeriod/1 -> Delay8/1, Delay2/1
  IfFinalState/1 -> Reset/2, OnlyAllowInNewPeriod/2, Reset1/2, T_count_switch/2, speed_old_switch/2, OR/2  "Allow_ToCheckOversampling"
  ABS/1 -> ProtectOverflow_rps/2, ProtectOverflow_T_count/2
  T_count_switch/1 -> ProtectOverflow_T_count/3, ABS/1
  Add2/1 -> speed_old_switch2/3
  Add1/1 -> speed_old_switch2/1
  Dir/1 -> speed_old_switch2/2
  Detec_edge/1 -> count_old1/1, reset_old_switch1/2  "pos and negative edges"
  reset_old1/1 -> Detec_edge/2, reset_old_switch1/3
  reset_old_switch1/1 -> reset_old1/1
  Encoder Line/1 -> Detec_edge/1, reset_old_switch1/1
  Constant3/1 -> ProtectToUseOmegaIfThetaJump1/2
  count_old1/1 -> ProtectToUseOmegaIfThetaJump1/1
  speed_old_switch2/1 -> T_count_switch/3, speed_old_switch/1
  T_count/1 -> Add1/1, Add2/1
  ProtectOverflow_T_count/1 -> T_count/1
  T/1 -> Add2/2, Add1/2
  speed_old/1 -> speed_old_switch/3
  speed_old_switch/1 -> speed_old/1, ProtectOverflow_rps/3
  Constant2/1 -> ProtectOverflow_rps/1
  Constant1/1 -> ProtectOverflow_T_count/1
  Constant/1 -> T_count_switch/1

== system gm_inc_enc_v26_vnl/Testfield/Counter_position_wOffset/Subsystem ==
  Add1 : Sum  AccumDataTypeStr=int16  OutDataTypeStr=int16
  Constant3 : Constant  Value=0  OutDataTypeStr=int16  SampleTime=-1
  Generate_Increment : Subsystem
  Resett_switch2 : Switch  Criteria=u2 ~= 0  OutDataTypeStr=int16  SaturateOnIntegerOverflow=off  InputSameDT=off
  reset_old6 : Delay  DelayLength=1
  speed_old_switch1 : Switch  Criteria=u2 ~= 0  SaturateOnIntegerOverflow=off  InputSameDT=off
  wires:
  speed_old_switch1/1 -> Add1/1
  Add1/1 -> Resett_switch2/3
  reset_old6/1 -> Resett_switch2/1
  ? -> Generate_Increment/1(Dir_in)
  Constant3/1 -> speed_old_switch1/3
  Resett_switch2/1 -> ?
  Generate_Increment/1(Increment) -> speed_old_switch1/1
  ? -> Add1/2
  ? -> reset_old6/1
  ? -> Resett_switch2/2
  ? -> speed_old_switch1/2

== system gm_inc_enc_v26_vnl/Create_Referenz/IncrementalEncoder_Floating/n_aus_theta_v4/Geschwindigkeitsfilter1 ==
  In1 : Inport
  Add1 : Sum  Inputs=+-
  Discrete-Time Integrator2 : DiscreteIntegrator  SampleTime=-1  ICPrevOutput=DiscIntNeverNeededParam  ICPrevScaledInput=DiscIntNeverNeededParam
  Gain2 2500 10000 : Gain  Gain=10000
  Scope1 : Scope  NumInputPorts=5
  Out1 : Outport  InitialOutput=[0]  VectorParamsAs1DForOutWhenUnconnected=off
  wires:
  Add1/1 -> Scope1/4, Gain2 2500 10000/1
  Gain2 2500 10000/1 -> Scope1/3, Discrete-Time Integrator2/1
  Discrete-Time Integrator2/1 -> Scope1/2, Out1/1, Add1/2
  In1/1 -> Scope1/5, Add1/1

== system gm_inc_enc_v26_vnl/IncEnc_V26/speed1/OS_factor_logic/align_oversamples ==
  oversampling_factor : Inport  OutDataTypeStr=uint16  PortDimensions=1  SampleTime=1e-08
  new_transition : Inport  Port=2  OutDataTypeStr=boolean  PortDimensions=[4]  SampleTime=1e-08
  states : Inport  Port=3  OutDataTypeStr=int16  PortDimensions=[4]  SampleTime=1e-08
  align_oversamples : MATLAB Function  TreatAsAtomicUnit=on
  delay_output : Outport  SampleTime=1e-08  VectorParamsAs1DForOutWhenUnconnected=off
  wires:
  align_oversamples/1(delay_output) -> delay_output/1
  states/1 -> align_oversamples/3(states)
  new_transition/1 -> align_oversamples/2(new_transition)
  oversampling_factor/1 -> align_oversamples/1(oversampling_factor)

== system gm_inc_enc_v26_vnl/IncEnc_V26/speed1/OS_factor_logic/oversample_factor ==
  AllowCheckOverSampl : Inport  OutDataTypeStr=boolean  PortDimensions=1  SampleTime=1e-08
  ReadBack_Omega : Inport  Port=2  OutDataTypeStr=fixdt(1, 24, 11)  PortDimensions=1  SampleTime=1e-08
  OverSamplOmega : Inport  Port=3  OutDataTypeStr=fixdt(1, 24, 11)  PortDimensions=1  SampleTime=1e-08
  state : Inport  Port=4  OutDataTypeStr=uint16  PortDimensions=1  SampleTime=1e-08
  InternalOmega : Inport  Port=5  OutDataTypeStr=fixdt(1, 24, 11)  PortDimensions=1  SampleTime=1e-08
  oversample_factor : MATLAB Function  TreatAsAtomicUnit=on
  state_Out : Outport  SampleTime=1e-08  VectorParamsAs1DForOutWhenUnconnected=off
  InternalOmega_Out : Outport  Port=2  SampleTime=1e-08  VectorParamsAs1DForOutWhenUnconnected=off
  wires:
  oversample_factor/2(InternalOmega_Out) -> InternalOmega_Out/1
  oversample_factor/1(state_Out) -> state_Out/1
  InternalOmega/1 -> oversample_factor/5(InternalOmega)
  state/1 -> oversample_factor/4(state)
  OverSamplOmega/1 -> oversample_factor/3(OverSamplOmega)
  ReadBack_Omega/1 -> oversample_factor/2(ReadBack_Omega)
  AllowCheckOverSampl/1 -> oversample_factor/1(AllowCheckOverSampl)

== system gm_inc_enc_v26_vnl/IncEnc_V26/speed1/calc_omega_instance1/invt_mult ==
  note: Invert 1/omega and muliply with synchronized oversampling factor
  New_Measurement : Inport  OutDataTypeStr=boolean  PortDimensions=1  SampleTime=1e-08
  rps : Inport  Port=2  OutDataTypeStr=fixdt(1, 38, 32)  PortDimensions=1  SampleTime=1e-08
  Oversampling Factor : Inport  Port=3  OutDataTypeStr=uint16  PortDimensions=1  SampleTime=1e-08
  Data Type Conversion2 : DataTypeConversion  OutDataTypeStr=fixdt(1, 24, 12)  SampleTime=1e-08  SaturateOnIntegerOverflow=off  RndMeth=Floor
  Data Type Conversion3 : DataTypeConversion  OutDataTypeStr=fixdt(0, 6, 0)  SampleTime=1e-08  SaturateOnIntegerOverflow=off  RndMeth=Floor
  Data Type Conversion4 : DataTypeConversion  OutDataTypeStr=fixdt(1, 32, 18)  SampleTime=1e-08  SaturateOnIntegerOverflow=off  RndMeth=Floor
  Div_i1 : Product  Inputs=**  OutDataTypeStr=fixdt(1, 30, 12)  SampleTime=1e-08
  Div_i1_out_dtc : DataTypeConversion  OutDataTypeStr=fixdt(1, 24, 11)  RndMeth=Simplest  SampleTime=1e-08
  HDL Reciprocal : Subsystem
  delayMatch : Delay  DelayLength=double(9)  InitialCondition=0  SampleTime=1e-08
  in_0_pipe : Delay  DelayLength=double(1)  InitialCondition=0  SampleTime=1e-08
  in_1_pipe : Delay  DelayLength=double(1)  InitialCondition=0  SampleTime=1e-08
  out_1_pipe : Delay  DelayLength=double(1)  InitialCondition=0  SampleTime=1e-08
  rd_{0..2,4} (4 alike) : Delay  DelayLength=double(1)  InitialCondition=0  SampleTime=1e-08
  rd_3 : Delay  DelayLength=double(8)  InitialCondition=0  SampleTime=1e-08
  omega_oversampled : Outport  SampleTime=1e-08
  New_Measurement_delayed : Outport  Port=2  SampleTime=1e-08
  wires:
  Data Type Conversion4/1 -> HDL Reciprocal/1(In1)
  rd_2/1 -> omega_oversampled/1
  delayMatch/1 -> New_Measurement_delayed/1
  HDL Reciprocal/1(Out1) -> rd_0/1
  New_Measurement/1 -> in_0_pipe/1
  rps/1 -> in_1_pipe/1
  Oversampling Factor/1 -> rd_1/1
  rd_0/1 -> Data Type Conversion2/1
  rd_1/1 -> Data Type Conversion3/1
  Div_i1_out_dtc/1 -> rd_2/1
  Data Type Conversion2/1 -> Div_i1/1
  Data Type Conversion3/1 -> rd_3/1
  rd_3/1 -> Div_i1/2
  Div_i1/1 -> rd_4/1
  rd_4/1 -> Div_i1_out_dtc/1
  in_0_pipe/1 -> out_1_pipe/1
  out_1_pipe/1 -> delayMatch/1
  in_1_pipe/1 -> Data Type Conversion4/1

== system gm_inc_enc_v26_vnl/IncEnc_V26/speed1/calc_omega_instance2/invt_mult ==
  note: Invert 1/omega and muliply with synchronized oversampling factor
  New_Measurement : Inport  OutDataTypeStr=boolean  PortDimensions=1  SampleTime=1e-08
  rps : Inport  Port=2  OutDataTypeStr=fixdt(1, 38, 32)  PortDimensions=1  SampleTime=1e-08
  Oversampling Factor : Inport  Port=3  OutDataTypeStr=uint16  PortDimensions=1  SampleTime=1e-08
  Data Type Conversion2 : DataTypeConversion  OutDataTypeStr=fixdt(1, 24, 12)  SampleTime=1e-08  SaturateOnIntegerOverflow=off  RndMeth=Floor
  Data Type Conversion3 : DataTypeConversion  OutDataTypeStr=fixdt(0, 6, 0)  SampleTime=1e-08  SaturateOnIntegerOverflow=off  RndMeth=Floor
  Data Type Conversion4 : DataTypeConversion  OutDataTypeStr=fixdt(1, 32, 18)  SampleTime=1e-08  SaturateOnIntegerOverflow=off  RndMeth=Floor
  Div_i1 : Product  Inputs=**  OutDataTypeStr=fixdt(1, 30, 12)  SampleTime=1e-08
  Div_i1_out_dtc : DataTypeConversion  OutDataTypeStr=fixdt(1, 24, 11)  RndMeth=Simplest  SampleTime=1e-08
  HDL Reciprocal : Subsystem
  delayMatch : Delay  DelayLength=double(9)  InitialCondition=0  SampleTime=1e-08
  in_0_pipe : Delay  DelayLength=double(1)  InitialCondition=0  SampleTime=1e-08
  in_1_pipe : Delay  DelayLength=double(1)  InitialCondition=0  SampleTime=1e-08
  out_1_pipe : Delay  DelayLength=double(1)  InitialCondition=0  SampleTime=1e-08
  rd_{0..2,4} (4 alike) : Delay  DelayLength=double(1)  InitialCondition=0  SampleTime=1e-08
  rd_3 : Delay  DelayLength=double(8)  InitialCondition=0  SampleTime=1e-08
  omega_oversampled : Outport  SampleTime=1e-08
  New_Measurement_delayed : Outport  Port=2  SampleTime=1e-08
  wires:
  Data Type Conversion4/1 -> HDL Reciprocal/1(In1)
  rd_2/1 -> omega_oversampled/1
  delayMatch/1 -> New_Measurement_delayed/1
  HDL Reciprocal/1(Out1) -> rd_0/1
  New_Measurement/1 -> in_0_pipe/1
  rps/1 -> in_1_pipe/1
  Oversampling Factor/1 -> rd_1/1
  rd_0/1 -> Data Type Conversion2/1
  rd_1/1 -> Data Type Conversion3/1
  Div_i1_out_dtc/1 -> rd_2/1
  Data Type Conversion2/1 -> Div_i1/1
  Data Type Conversion3/1 -> rd_3/1
  rd_3/1 -> Div_i1/2
  Div_i1/1 -> rd_4/1
  rd_4/1 -> Div_i1_out_dtc/1
  in_0_pipe/1 -> out_1_pipe/1
  out_1_pipe/1 -> delayMatch/1
  in_1_pipe/1 -> Data Type Conversion4/1

== system gm_inc_enc_v26_vnl/IncEnc_V26/speed1/calc_omega_instance3/invt_mult ==
  note: Invert 1/omega and muliply with synchronized oversampling factor
  New_Measurement : Inport  OutDataTypeStr=boolean  PortDimensions=1  SampleTime=1e-08
  rps : Inport  Port=2  OutDataTypeStr=fixdt(1, 38, 32)  PortDimensions=1  SampleTime=1e-08
  Oversampling Factor : Inport  Port=3  OutDataTypeStr=uint16  PortDimensions=1  SampleTime=1e-08
  Data Type Conversion2 : DataTypeConversion  OutDataTypeStr=fixdt(1, 24, 12)  SampleTime=1e-08  SaturateOnIntegerOverflow=off  RndMeth=Floor
  Data Type Conversion3 : DataTypeConversion  OutDataTypeStr=fixdt(0, 6, 0)  SampleTime=1e-08  SaturateOnIntegerOverflow=off  RndMeth=Floor
  Data Type Conversion4 : DataTypeConversion  OutDataTypeStr=fixdt(1, 32, 18)  SampleTime=1e-08  SaturateOnIntegerOverflow=off  RndMeth=Floor
  Div_i1 : Product  Inputs=**  OutDataTypeStr=fixdt(1, 30, 12)  SampleTime=1e-08
  Div_i1_out_dtc : DataTypeConversion  OutDataTypeStr=fixdt(1, 24, 11)  RndMeth=Simplest  SampleTime=1e-08
  HDL Reciprocal : Subsystem
  delayMatch : Delay  DelayLength=double(9)  InitialCondition=0  SampleTime=1e-08
  in_0_pipe : Delay  DelayLength=double(1)  InitialCondition=0  SampleTime=1e-08
  in_1_pipe : Delay  DelayLength=double(1)  InitialCondition=0  SampleTime=1e-08
  out_1_pipe : Delay  DelayLength=double(1)  InitialCondition=0  SampleTime=1e-08
  rd_{0..2,4} (4 alike) : Delay  DelayLength=double(1)  InitialCondition=0  SampleTime=1e-08
  rd_3 : Delay  DelayLength=double(8)  InitialCondition=0  SampleTime=1e-08
  omega_oversampled : Outport  SampleTime=1e-08
  New_Measurement_delayed : Outport  Port=2  SampleTime=1e-08
  wires:
  Data Type Conversion4/1 -> HDL Reciprocal/1(In1)
  rd_2/1 -> omega_oversampled/1
  delayMatch/1 -> New_Measurement_delayed/1
  HDL Reciprocal/1(Out1) -> rd_0/1
  New_Measurement/1 -> in_0_pipe/1
  rps/1 -> in_1_pipe/1
  Oversampling Factor/1 -> rd_1/1
  rd_0/1 -> Data Type Conversion2/1
  rd_1/1 -> Data Type Conversion3/1
  Div_i1_out_dtc/1 -> rd_2/1
  Data Type Conversion2/1 -> Div_i1/1
  Data Type Conversion3/1 -> rd_3/1
  rd_3/1 -> Div_i1/2
  Div_i1/1 -> rd_4/1
  rd_4/1 -> Div_i1_out_dtc/1
  in_0_pipe/1 -> out_1_pipe/1
  out_1_pipe/1 -> delayMatch/1
  in_1_pipe/1 -> Data Type Conversion4/1
